simulink model "Speed_Control_Of_BLDC"  (R2024a)
settings: Solver=VariableStepAuto  StartTime=0.0  StopTime=14  RelTol=1e-3
libraries: simulink x7, spsMosfetLib x6, spsVoltageMeasurementLib x3, spsControlledVoltageSourceLib x1, spsGroundLib x1, slpidlib x1, sps_lib x1
settings Model: Creator=net  LastModifiedBy=Anjali Sharma
settings SolverCC: AlgebraicLoopSolver=TrustRegion
settings DataIOCC: ReturnWorkspaceOutputs=off
settings OptimizationCC: ReuseModelBlockBuffer=off
settings DebuggingCC: UnconnectedInputMsg=warning  UnconnectedOutputMsg=warning  UnconnectedLineMsg=warning  ArithmeticOperatorsInVariantConditions=warning
settings ModelReferenceCC: EnableRefExpFcnMdlSchedulingChecks=on
settings SFSimCC: SimUseLocalCustomCode=off  CustomCodeUndefinedFunction=UseInterfaceOnly
settings RTWCC: RTWUseLocalCustomCode=off  GPUComputeCapability=3.5
settings CodeAppCC: StateflowObjectComments=on
settings SimscapeCC: SimscapeNormalizeSystem=off

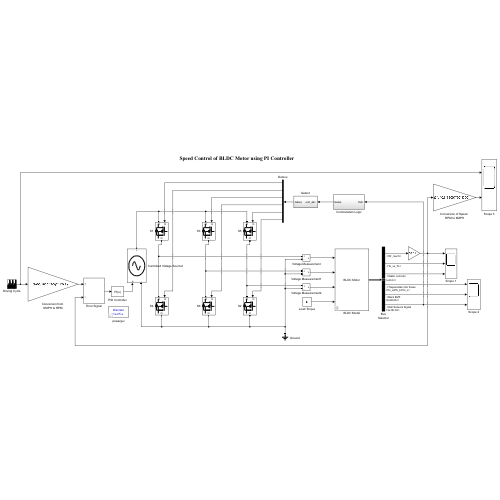
[thumbnail: Simulink's stored preview of the top-level diagram]
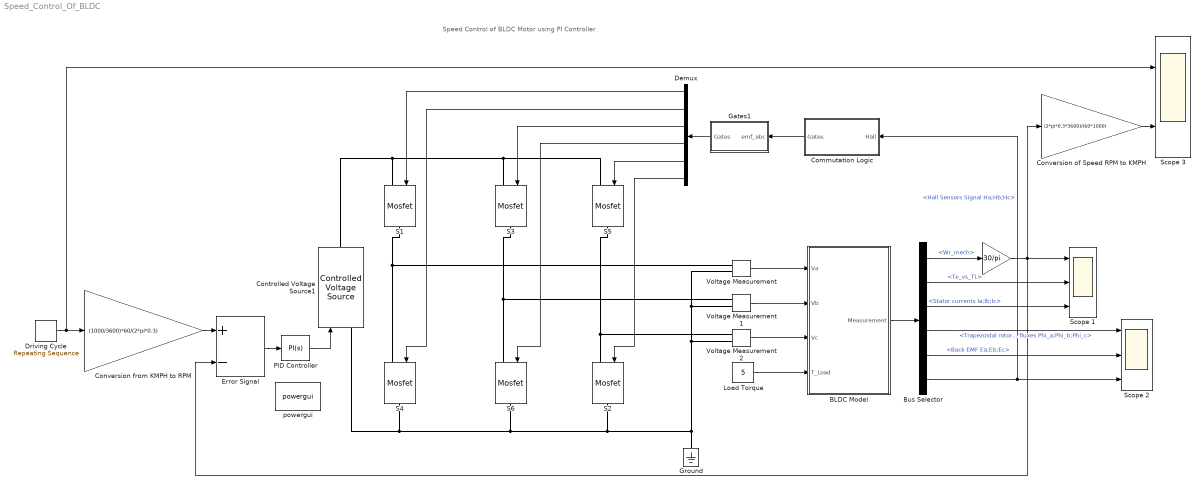
== system Speed_Control_Of_BLDC ==
  note: Speed Control of BLDC Motor using PI Controller
  " " : Gain  Gain=30/pi  SaturateOnIntegerOverflow=on  OutDataTypeStr=Inherit: Same as input  ParamDataTypeStr=Inherit: Same as input
  BLDC Model : Subsystem  mask(BLDC Motor :){Rs=1.43, Lls=9.4e-3, Phi_m=0.2158, J=5.5e-3, B=2e-3, P=4}
      mask prompts: Rs "Resistance - Rs [ohms]"; Lls "Inductance - Lls [H]"; Phi_m "Rotor Flux [wb]"; J "Rotor Inertia - J [kg-m^2]"; B "Friction Coefficient -B"; P "No of Poles"
      mask init:
      | Trap=0.5;
      mask Display: fprintf('BLDC Motor')
  Bus Selector : BusSelector  OutputSignals=|
      | Wr_mech,Te_vs_TL,Stator currents
      | Ia;Ib;Ic,Trapezoidal rotor fluxes
      | Phi_a;Phi_b;Phi_c,Back EMF
      | Ea;Eb;Ec,Hall Sensors Signal
      | Ha;Hb;Hc
  Commutation Logic : Subsystem
  Controlled Voltage Source1 : spsControlledVoltageSourceLib/Controlled Voltage Source  Initialize=on  Source_Type=AC  Amplitude=100  Phase=0  Frequency=0  Measurements=None
  "Conversion from KMPH to RPM " : Gain  Gain=(1000/3600)*60/(2*pi*0.3)
  Conversion of Speed RPM to KMPH : Gain  Gain=(2*pi*0.3*3600)/(60*1000)  SaturateOnIntegerOverflow=on  OutDataTypeStr=Inherit: Same as input  ParamDataTypeStr=Inherit: Same as input
  Demux : Demux  Outputs=6
  Driving Cycle : simulink/Sources/Repeating Sequence  rep_seq_t=[0 1 2 3 4 5 6 7 8 9 10 11 11.0001 12 13]  rep_seq_y=[0 0 20 20 0 0 30 30 0 0 50 50 40 40 0]
  Error Signal : Sum  Inputs=+-
  Gates1 : Subsystem
  Ground : spsGroundLib/Ground  LConnTagsString=a
  Load Torque : Constant  Value=5
  PID Controller : slpidlib/PID Controller  Controller=PI  Form=Parallel  TimeDomain=Continuous-time  UseExternalTs=off  SampleTime=-1  IntegratorMethod=Forward Euler  FilterMethod=Forward Euler  ControllerParametersSource=internal  P=0.754336715688095  I=49.9879440674314  UseKiTs=off  D=0.00192762182262476  UseExternalDerivativeSource=off  N=289.099868323626  UseFilter=on  TunerSelectOption=Transfer Function Based (PID Tuner App)  InitialConditionSource=internal  InitialConditionForIntegrator=0  InitialConditionForFilter=0  DifferentiatorICPrevScaledInput=0  ExternalReset=none  TrackingMode=off  Kt=1  LimitOutput=off  SatLimitsSource=internal  UpperSaturationLimit=inf  LowerSaturationLimit=-inf  LinearizeAsGain=on  AntiWindupMode=none  Kb=1  LimitIntegrator=off  UpperIntegratorSaturationLimit=inf  LowerIntegratorSaturationLimit=-inf  POutMin=[]  POutMax=[]  IOutMin=[]  IOutMax=[]  DOutMin=[]  DOutMax=[]  NOutMin=[]  NOutMax=[]  SumOutMin=[]  SumOutMax=[]  SaturationOutMin=[]  SaturationOutMax=[]  PParamMin=[]  PParamMax=[]  IParamMin=[]  IParamMax=[]  DParamMin=[]  DParamMax=[]  NParamMin=[]  NParamMax=[]  KbParamMin=[]  KbParamMax=[]  KtParamMin=[]  KtParamMax=[]  KbOutMin=[]  KbOutMax=[]  KtOutMin=[]  KtOutMax=[]  IntegratorOutMin=[]  IntegratorOutMax=[]  FilterOutMin=[]  FilterOutMax=[]  SumI1OutMin=[]  SumI1OutMax=[]  SumI2OutMin=[]  SumI2OutMax=[]  SumI3OutMin=[]  SumI3OutMax=[]  SumI4OutMin=[]  SumI4OutMax=[]  SumDOutMin=[]  SumDOutMax=[]  DifferentiatorOutMin=[]  DifferentiatorOutMax=[]  FilterDiffOutCoefMin=[]  FilterDiffOutCoefMax=[]  ReciprocalOutMin=[]  ReciprocalOutMax=[]  SumDenOutMin=[]  SumDenOutMax=[]  SumNumOutMin=[]  SumNumOutMax=[]  DivideOutMin=[]  DivideOutMax=[]  UdiffTsProdOutMin=[]  UdiffTsProdOutMax=[]  NTsProdOutMin=[]  NTsProdOutMax=[]  UintegralTsProdOutMin=[]  UintegralTsProdOutMax=[]  UngainTsProdOutMin=[]  UngainTsProdOutMax=[]  ClampingZeroOutDataTypeStr=Inherit: Inherit via back propagation  ClampingZeroOutMin=[]  ClampingZeroOutMax=[]  FilterDenConstantOutDataTypeStr=Inherit: Inherit via back propagation  FilterDenConstantOutMin=[]  FilterDenConstantOutMax=[]  PCopyOutDataTypeStr=Inherit: Inherit via back propagation  PCopyOutMin=[]  PCopyOutMax=[]  NCopyOutDataTypeStr=Inherit: Inherit via back propagation  NCopyOutMin=[]  NCopyOutMax=[]  IntegratorContinuousStateAttributes=''  IntegratorStateMustResolveToSignalObject=off  IntegratorRTWStateStorageClass=Auto  FilterContinuousStateAttributes=''  FilterStateMustResolveToSignalObject=off  FilterRTWStateStorageClass=Auto  ParallelPVariant=InternalParameters  IdealPVariant=Disabled  IVariant=InternalParameters  DVariant=Disabled  IntegratorVariant=Continuous  SatVariant=Disabled  AWVariant=Passthrough  PCopyVariant=Disabled  TRVariant=Disabled  FdbkBlocksVariant=Forward  IdealPFdbkVariant=Disabled  SatFdbkVariant=Disabled  DerivativeFilterVariant=Disabled  NVariant=Disabled  NCopyVariant=Disabled_SignalSpec  FilterICVariant=Disabled  IntegratorICVariant=InternalICs  ExternalResetVariant=Disabled  TRSumVariant=Passthrough  SumFdbkVariant=Disabled  SumVariant=Sum_PI  TsampFilterVariant=InternalTs  TsampNgainVariant=Passthrough  TsampIntegralVariant=Disabled_SignalSpec  ExternalSaturationOutDataTypeStr=Inherit: Same as second input  DerivativeSourceVariant=Disabled
  S{1..6} (6 alike) : spsMosfetLib/Mosfet  Ron=0.1  Lon=0  Rd=0.01  Vfd=0  IC=0  Rs=1e5  Cs=inf  Measurements=off
  Scope 1 : Scope  NumInputPorts=3
  Scope 2 : Scope  NumInputPorts=3
  Scope 3 : Scope  NumInputPorts=2
  Voltage Measurement : spsVoltageMeasurementLib/Voltage Measurement  PhasorSimulation=off  OutputType=Complex  PSBequivalent=0
  Voltage Measurement1 : spsVoltageMeasurementLib/Voltage Measurement  PhasorSimulation=off  OutputType=Complex  PSBequivalent=0
  Voltage Measurement2 : spsVoltageMeasurementLib/Voltage Measurement  PhasorSimulation=off  OutputType=Complex  PSBequivalent=0
  powergui : sps_lib/powergui  Priority=1  SimulationMode=Discrete  SampleTime=50e-6  frequency=60  Iterations=50  frequencyindice=0  Pbase=100e6  ErrMax=1e-4  UnitsV=kV  UnitsW=MW  buscounter=0  FunctionMessages=off  echomessages=off  EnableUseOfTLC=off  CurrentSourceSwitches=off  DisableSnubberDevices=off  DisableRonSwitches=off  DisableVfSwitches=off  DisplayEquations=off  AutomaticDiscreteSolvers=off  SolverType=Tustin/Backward Euler (TBE)  Interpol=off  ExternalGateDelay=off  methode=off  Ts=10  x0status=blocks  SPID=off  SwTol=0  HookPort=off  NonlinearTolerance=1e-4  nMaxIteration=100  ContinueOnMaxIteration=off  RestoreLinks=warning  ResistiveCurrentMeasurement=off  Frange=[0:2:500]  Ylog=off  Xlog=on  ShowGrid=off  save=off  variable=ZData  structure=0  ZoomFFT=off  StartTime=0.0  cycles=1  DisplayStyle=1  fundamental=60  FreqAxis=off  MaxFrequency=1000  frequencyindicesteady=1  RmsSteady=1  display=off
  wires:
  Voltage Measurement/1 -> BLDC Model/1(Va)
  Voltage Measurement1/1 -> BLDC Model/2(Vb)
  Voltage Measurement2/1 -> BLDC Model/3(Vc)
  Commutation Logic/1(Gates) -> Gates1/1("emf_abc ")
  Load Torque/1 -> BLDC Model/4(T_Load)
  Gates1/1(Gates) -> Demux/1
  Demux/1 -> S1/1
  Demux/2 -> S4/1
  Demux/3 -> S3/1
  Demux/5 -> S5/1
  Demux/4 -> S6/1
  Demux/6 -> S2/1
  Error Signal/1 -> PID Controller/1
  PID Controller/1 -> Controlled Voltage Source1/1
  BLDC Model/1(Measurement) -> Bus Selector/1
  Bus Selector/6 -> Scope 2/3, Commutation Logic/1("Hall ")  "<Hall Sensors Signal Ha;Hb;Hc>"
  Bus Selector/4 -> Scope 2/1  "<Trapezoidal rotor fluxes Phi_a;Phi_b;Phi_c>"
  Bus Selector/3 -> Scope 1/3  "<Stator currents Ia;Ib;Ic>"
  Bus Selector/2 -> Scope 1/2  "<Te_vs_TL>"
  Bus Selector/5 -> Scope 2/2  "<Back EMF Ea;Eb;Ec>"
  Bus Selector/1 -> " "/1  "<Wr_mech>"
  " "/1 -> Scope 1/1, Error Signal/2, Conversion of Speed RPM to KMPH/1
  "Conversion from KMPH to RPM "/1 -> Error Signal/1
  Driving Cycle/1 -> Scope 3/1, "Conversion from KMPH to RPM "/1
  Conversion of Speed RPM to KMPH/1 -> Scope 3/2
  connections:
  S5/LConn1 -- S3/LConn1 -- S1/LConn1 -- Controlled Voltage Source1/RConn1
  Voltage Measurement/LConn2 -- Voltage Measurement1/LConn2 -- Voltage Measurement2/LConn2 -- Ground/LConn1 -- S2/RConn1 -- S4/RConn1 -- Controlled Voltage Source1/LConn1 -- S6/RConn1
  S1/RConn1 -- S4/LConn1 -- Voltage Measurement/LConn1
  S3/RConn1 -- S6/LConn1 -- Voltage Measurement1/LConn1
  S5/RConn1 -- S2/LConn1 -- Voltage Measurement2/LConn1

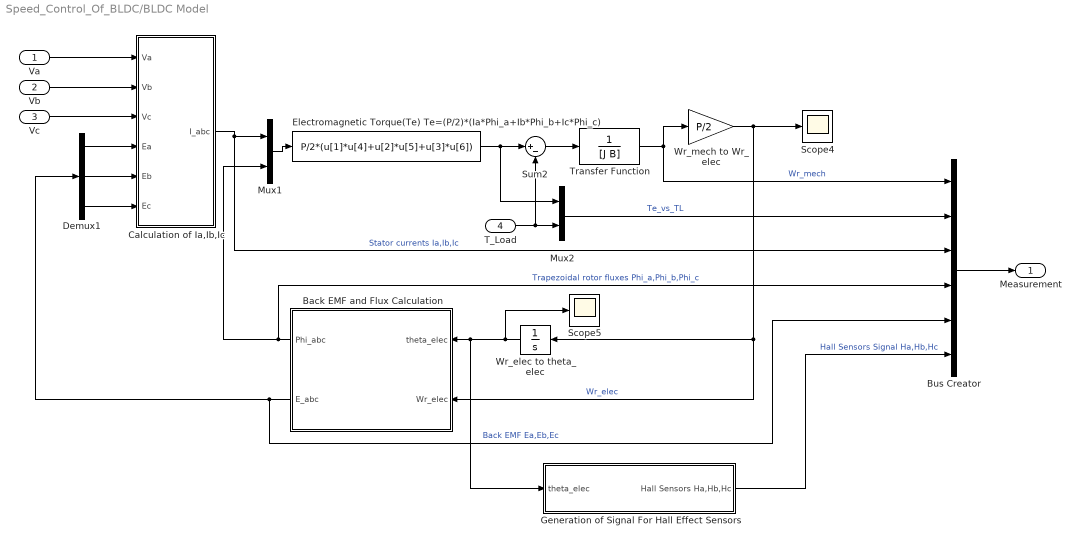
== system Speed_Control_Of_BLDC/BLDC Model ==
  Va : Inport
  Vb : Inport  Port=2
  Vc : Inport  Port=3
  T_Load : Inport  Port=4
  Back EMF and Flux Calculation : Subsystem
  Bus Creator : BusCreator  Inputs=6
  Calculation of Ia,Ib,Ic : Subsystem
  Demux1 : Demux  Outputs=3
  Electromagnetic Torque(Te) Te=(P/2)*(Ia*Phi_a+Ib*Phi_b+Ic*Phi_c) : Fcn  Expr=P/2*(u[1]*u[4]+u[2]*u[5]+u[3]*u[6])
  Generation of Signal For Hall Effect Sensors : Subsystem
  Mux1 : Mux  Inputs=2
  Mux2 : Mux  Inputs=2
  Scope4 : Scope
  Scope5 : Scope
  Sum2 : Sum  Inputs=|+-
  Transfer Function : TransferFcn  Denominator=[J B]
  Wr_elec to theta_elec : Integrator
  Wr_mech to Wr_elec : Gain  Gain=P/2
  Measurement : Outport
  wires:
  Vc/1 -> Calculation of Ia,Ib,Ic/3(Vc)
  Va/1 -> Calculation of Ia,Ib,Ic/1(Va)
  Vb/1 -> Calculation of Ia,Ib,Ic/2(Vb)
  Sum2/1 -> Transfer Function/1
  Mux1/1 -> Electromagnetic Torque(Te) Te=(P/2)*(Ia*Phi_a+Ib*Phi_b+Ic*Phi_c)/1
  Demux1/3 -> Calculation of Ia,Ib,Ic/6(Ec)
  Demux1/2 -> Calculation of Ia,Ib,Ic/5(Eb)
  Demux1/1 -> Calculation of Ia,Ib,Ic/4(Ea)
  Wr_elec to theta_elec/1 -> Generation of Signal For Hall Effect Sensors/1(theta_elec), Back EMF and Flux Calculation/1(theta_elec), Scope5/1
  Bus Creator/1 -> Measurement/1
  Transfer Function/1 -> Wr_mech to Wr_elec/1, Bus Creator/1  "Wr_mech"
  Back EMF and Flux Calculation/2(E_abc) -> Bus Creator/5, Demux1/1  "Back EMF Ea,Eb,Ec"
  Wr_mech to Wr_elec/1 -> Back EMF and Flux Calculation/2(Wr_elec), Wr_elec to theta_elec/1, Scope4/1  "Wr_elec"
  Back EMF and Flux Calculation/1(Phi_abc) -> Mux1/2, Bus Creator/4  "Trapezoidal rotor fluxes Phi_a,Phi_b,Phi_c"
  Calculation of Ia,Ib,Ic/1(I_abc) -> Bus Creator/3, Mux1/1  "Stator currents Ia,Ib,Ic"
  Electromagnetic Torque(Te) Te=(P/2)*(Ia*Phi_a+Ib*Phi_b+Ic*Phi_c)/1 -> Mux2/1, Sum2/1
  Generation of Signal For Hall Effect Sensors/1(Hall Sensors Ha,Hb,Hc) -> Bus Creator/6  "Hall Sensors Signal Ha,Hb,Hc"
  Mux2/1 -> Bus Creator/2  "Te_vs_TL"
  T_Load/1 -> Sum2/2, Mux2/2

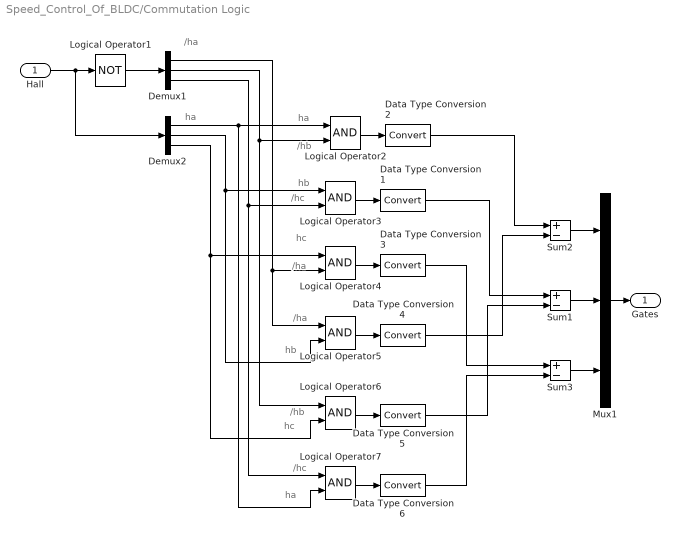
== system Speed_Control_Of_BLDC/Commutation Logic ==
  note: ha
  note: /hc
  note: hc
  note: /hb
  note: hb
  note: /ha
  note: /ha
  note: hc
  note: /hc
  note: hb
  note: /hb
  note: ha
  note: ha
  note: /ha
  "Hall " : Inport
  Data Type Conversion{1..6} (6 alike) : DataTypeConversion  SaturateOnIntegerOverflow=off  RndMeth=Floor
  Demux1 : Demux  Outputs=3
  Demux2 : Demux  Outputs=3
  Logical Operator1 : Logic  Operator=NOT  AllPortsSameDT=off  OutDataTypeStr=boolean
  Logical Operator{2..7} (6 alike) : Logic  AllPortsSameDT=off  OutDataTypeStr=boolean
  Mux1 : Mux  Inputs=3
  Sum1 : Sum  Inputs=+-  OutDataTypeStr=double
  Sum2 : Sum  Inputs=+-  OutDataTypeStr=double
  Sum3 : Sum  Inputs=+-  OutDataTypeStr=double
  Gates : Outport
  wires:
  Demux2/3 -> Logical Operator6/2, Logical Operator4/1
  Sum2/1 -> Mux1/1
  Mux1/1 -> Gates/1
  Logical Operator1/1 -> Demux1/1
  Logical Operator7/1 -> Data Type Conversion6/1
  Sum3/1 -> Mux1/3
  Logical Operator4/1 -> Data Type Conversion3/1
  Data Type Conversion4/1 -> Sum2/2
  Data Type Conversion5/1 -> Sum1/2
  Demux1/1 -> Logical Operator5/1, Logical Operator4/2
  Data Type Conversion3/1 -> Sum3/1
  Data Type Conversion6/1 -> Sum3/2
  Logical Operator5/1 -> Data Type Conversion4/1
  Data Type Conversion2/1 -> Sum2/1
  Logical Operator6/1 -> Data Type Conversion5/1
  Demux1/2 -> Logical Operator2/2, Logical Operator6/1
  Logical Operator2/1 -> Data Type Conversion2/1
  Logical Operator3/1 -> Data Type Conversion1/1
  "Hall "/1 -> Demux2/1, Logical Operator1/1
  Data Type Conversion1/1 -> Sum1/1
  Sum1/1 -> Mux1/2
  Demux2/2 -> Logical Operator5/2, Logical Operator3/1
  Demux1/3 -> Logical Operator3/2, Logical Operator7/1
  Demux2/1 -> Logical Operator2/1, Logical Operator7/2

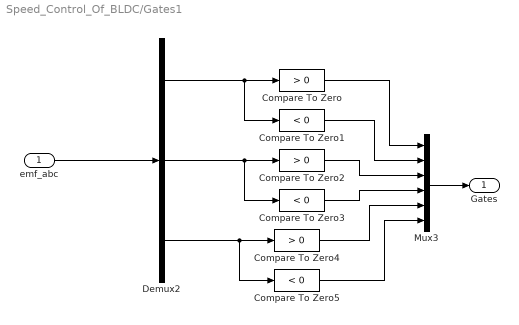
== system Speed_Control_Of_BLDC/Gates1 ==
  "emf_abc " : Inport
  Compare To Zero : simulink/Logic and Bit Operations/Compare To Zero  relop=>  OutDataTypeStr=boolean  ZeroCross=off
  Compare To Zero1 : simulink/Logic and Bit Operations/Compare To Zero  relop=<  OutDataTypeStr=boolean  ZeroCross=off
  Compare To Zero2 : simulink/Logic and Bit Operations/Compare To Zero  relop=>  OutDataTypeStr=boolean  ZeroCross=off
  Compare To Zero3 : simulink/Logic and Bit Operations/Compare To Zero  relop=<  OutDataTypeStr=boolean  ZeroCross=off
  Compare To Zero4 : simulink/Logic and Bit Operations/Compare To Zero  relop=>  OutDataTypeStr=boolean  ZeroCross=off
  Compare To Zero5 : simulink/Logic and Bit Operations/Compare To Zero  relop=<  OutDataTypeStr=boolean  ZeroCross=off
  Demux2 : Demux  Outputs=3
  Mux3 : Mux  Inputs=6
  Gates : Outport
  wires:
  "emf_abc "/1 -> Demux2/1
  Mux3/1 -> Gates/1
  Demux2/1 -> Compare To Zero/1, Compare To Zero1/1
  Demux2/2 -> Compare To Zero2/1, Compare To Zero3/1
  Demux2/3 -> Compare To Zero4/1, Compare To Zero5/1
  Compare To Zero/1 -> Mux3/1
  Compare To Zero1/1 -> Mux3/2
  Compare To Zero2/1 -> Mux3/3
  Compare To Zero3/1 -> Mux3/4
  Compare To Zero4/1 -> Mux3/5
  Compare To Zero5/1 -> Mux3/6

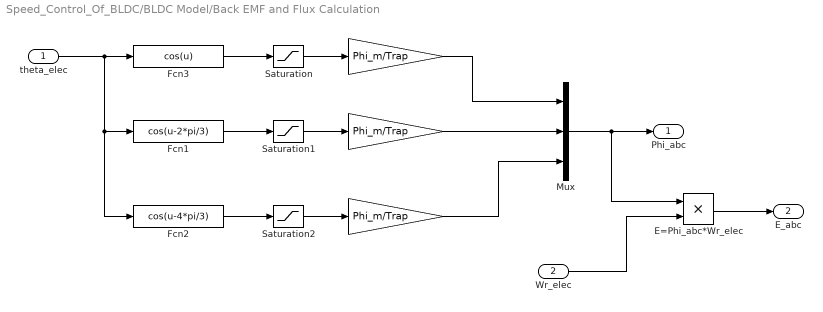
== system Speed_Control_Of_BLDC/BLDC Model/Back EMF and Flux Calculation ==
  theta_elec : Inport
  Wr_elec : Inport  Port=2
  " " : Gain  Gain=Phi_m/Trap
  " " : Gain  Gain=Phi_m/Trap
  " " : Gain  Gain=Phi_m/Trap
  E=Phi_abc*Wr_elec : Product
  Fcn1 : Fcn  Expr=cos(u-2*pi/3)
  Fcn2 : Fcn  Expr=cos(u-4*pi/3)
  Fcn3 : Fcn  Expr=cos(u)
  Mux : Mux  Inputs=3
  Saturation : Saturate  UpperLimit=Trap  LowerLimit=-Trap
  Saturation1 : Saturate  UpperLimit=Trap  LowerLimit=-Trap
  Saturation2 : Saturate  UpperLimit=Trap  LowerLimit=-Trap
  Phi_abc : Outport
  E_abc : Outport  Port=2
  wires:
  Fcn3/1 -> Saturation/1
  theta_elec/1 -> Fcn2/1, Fcn1/1, Fcn3/1
  Fcn2/1 -> Saturation2/1
  Fcn1/1 -> Saturation1/1
  " "/1 -> Mux/1
  " "/1 -> Mux/2
  " "/1 -> Mux/3
  Mux/1 -> Phi_abc/1, E=Phi_abc*Wr_elec/1
  Wr_elec/1 -> E=Phi_abc*Wr_elec/2
  E=Phi_abc*Wr_elec/1 -> E_abc/1
  Saturation/1 -> " "/1
  Saturation1/1 -> " "/1
  Saturation2/1 -> " "/1

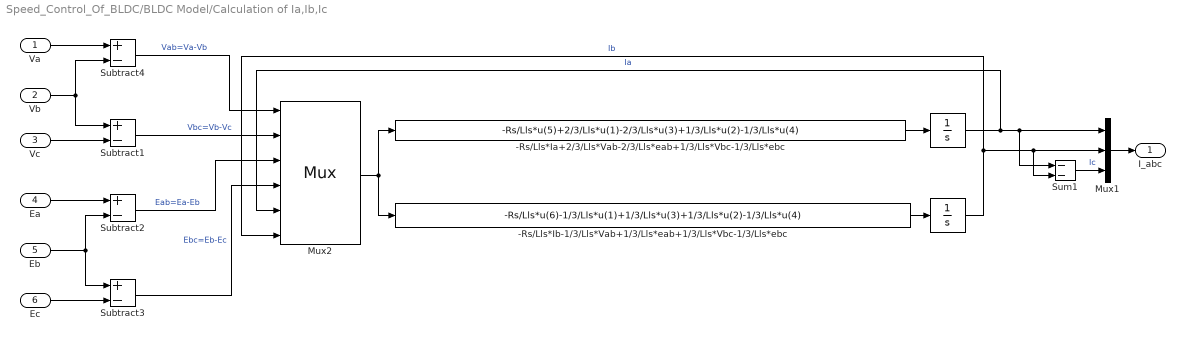
== system Speed_Control_Of_BLDC/BLDC Model/Calculation of Ia,Ib,Ic ==
  Va : Inport
  Vb : Inport  Port=2
  Vc : Inport  Port=3
  Ea : Inport  Port=4
  Eb : Inport  Port=5
  Ec : Inport  Port=6
  " " : Integrator
  " " : Integrator
  -Rs/Lls*Ia+2/3/Lls*Vab-2/3/Lls*eab+1/3/Lls*Vbc-1/3/Lls*ebc : Fcn  Expr=-Rs/Lls*u(5)+2/3/Lls*u(1)-2/3/Lls*u(3)+1/3/Lls*u(2)-1/3/Lls*u(4)
  -Rs/Lls*Ib-1/3/Lls*Vab+1/3/Lls*eab+1/3/Lls*Vbc-1/3/Lls*ebc : Fcn  Expr=-Rs/Lls*u(6)-1/3/Lls*u(1)+1/3/Lls*u(3)+1/3/Lls*u(2)-1/3/Lls*u(4)
  Mux1 : Mux  Inputs=3
  Mux2 : Mux  Inputs=6
      settings: DisplayOption=signals
  Subtract{1..4} (4 alike) : Sum  Inputs=+-
  Sum1 : Sum  Inputs=--  SaturateOnIntegerOverflow=on
  I_abc : Outport
  wires:
  Va/1 -> Subtract4/1
  Vb/1 -> Subtract4/2, Subtract1/1
  Vc/1 -> Subtract1/2
  Eb/1 -> Subtract3/1, Subtract2/2
  Ea/1 -> Subtract2/1
  Ec/1 -> Subtract3/2
  -Rs/Lls*Ia+2/3/Lls*Vab-2/3/Lls*eab+1/3/Lls*Vbc-1/3/Lls*ebc/1 -> " "/1
  Subtract3/1 -> Mux2/4  "Ebc=Eb-Ec"
  -Rs/Lls*Ib-1/3/Lls*Vab+1/3/Lls*eab+1/3/Lls*Vbc-1/3/Lls*ebc/1 -> " "/1
  Subtract4/1 -> Mux2/1  "Vab=Va-Vb"
  Subtract1/1 -> Mux2/2  "Vbc=Vb-Vc"
  Subtract2/1 -> Mux2/3  "Eab=Ea-Eb"
  Mux2/1 -> -Rs/Lls*Ia+2/3/Lls*Vab-2/3/Lls*eab+1/3/Lls*Vbc-1/3/Lls*ebc/1, -Rs/Lls*Ib-1/3/Lls*Vab+1/3/Lls*eab+1/3/Lls*Vbc-1/3/Lls*ebc/1
  " "/1 -> Mux1/2, Sum1/2, Mux2/6  "Ib"
  " "/1 -> Sum1/1, Mux1/1, Mux2/5  "Ia"
  Sum1/1 -> Mux1/3  "Ic"
  Mux1/1 -> I_abc/1

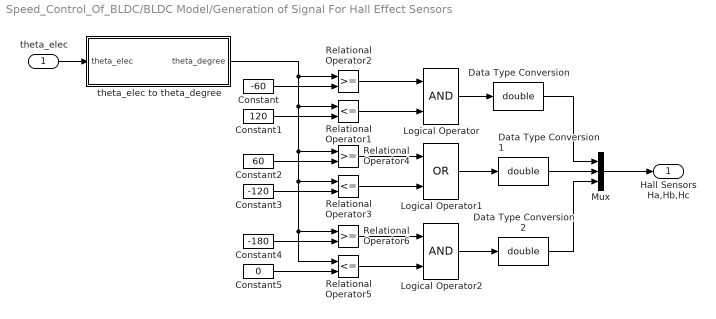
== system Speed_Control_Of_BLDC/BLDC Model/Generation of Signal For Hall Effect Sensors ==
  theta_elec : Inport
  Constant : Constant  Value=-60
  Constant1 : Constant  Value=120
  Constant2 : Constant  Value=60
  Constant3 : Constant  Value=-120
  Constant4 : Constant  Value=-180
  Constant5 : Constant  Value=0
  Data Type Conversion : DataTypeConversion  OutDataTypeStr=double
  Data Type Conversion1 : DataTypeConversion  OutDataTypeStr=double
  Data Type Conversion2 : DataTypeConversion  OutDataTypeStr=double
  Logical Operator : Logic  AllPortsSameDT=off  OutDataTypeStr=boolean
  Logical Operator1 : Logic  Operator=OR  AllPortsSameDT=off  OutDataTypeStr=boolean
  Logical Operator2 : Logic  AllPortsSameDT=off  OutDataTypeStr=boolean
  Mux : Mux  Inputs=3
  Relational Operator1 : RelationalOperator  Operator=<=
  Relational Operator2 : RelationalOperator
  Relational Operator3 : RelationalOperator  Operator=<=
  Relational Operator4 : RelationalOperator
  Relational Operator5 : RelationalOperator  Operator=<=
  Relational Operator6 : RelationalOperator
  theta_elec to theta_degree : Subsystem
  Hall Sensors Ha,Hb,Hc : Outport
  wires:
  Constant3/1 -> Relational Operator3/2
  Data Type Conversion2/1 -> Mux/3
  Data Type Conversion1/1 -> Mux/2
  Data Type Conversion/1 -> Mux/1
  Relational Operator5/1 -> Logical Operator2/2
  Logical Operator2/1 -> Data Type Conversion2/1
  Relational Operator6/1 -> Logical Operator2/1
  Constant4/1 -> Relational Operator6/2
  Constant5/1 -> Relational Operator5/2
  Relational Operator3/1 -> Logical Operator1/2
  Logical Operator1/1 -> Data Type Conversion1/1
  Logical Operator/1 -> Data Type Conversion/1
  Mux/1 -> Hall Sensors Ha,Hb,Hc/1
  Relational Operator2/1 -> Logical Operator/1
  Relational Operator1/1 -> Logical Operator/2
  theta_elec to theta_degree/1(theta_degree) -> Relational Operator4/1, Relational Operator3/1, Relational Operator5/1, Relational Operator6/1, Relational Operator1/1, Relational Operator2/1
  Constant/1 -> Relational Operator2/2
  Relational Operator4/1 -> Logical Operator1/1
  Constant1/1 -> Relational Operator1/2
  Constant2/1 -> Relational Operator4/2
  theta_elec/1 -> theta_elec to theta_degree/1(theta_elec)

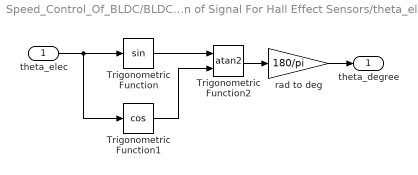
== system Speed_Control_Of_BLDC/BLDC Model/Generation of Signal For Hall Effect Sensors/theta_elec to theta_degree ==
  theta_elec : Inport
  Trigonometric Function : Trigonometry
  Trigonometric Function1 : Trigonometry  Operator=cos
  Trigonometric Function2 : Trigonometry  Operator=atan2
  rad to deg : Gain  Gain=180/pi  SaturateOnIntegerOverflow=on  OutDataTypeStr=Inherit: Same as input  ParamDataTypeStr=Inherit: Same as input
  theta_degree : Outport
  wires:
  Trigonometric Function2/1 -> rad to deg/1
  Trigonometric Function/1 -> Trigonometric Function2/1
  Trigonometric Function1/1 -> Trigonometric Function2/2
  theta_elec/1 -> Trigonometric Function1/1, Trigonometric Function/1
  rad to deg/1 -> theta_degree/1
